simulink library "MBDS_Applications"  (R2018b)
settings: Solver=ode45  StartTime=0.0  StopTime=10.0  RelTol=1e-3
undefined symbols (not defined in the file or in its folder): Ts
libraries: KIBES_Signal x297, simulink x7
(part 4 of 6)

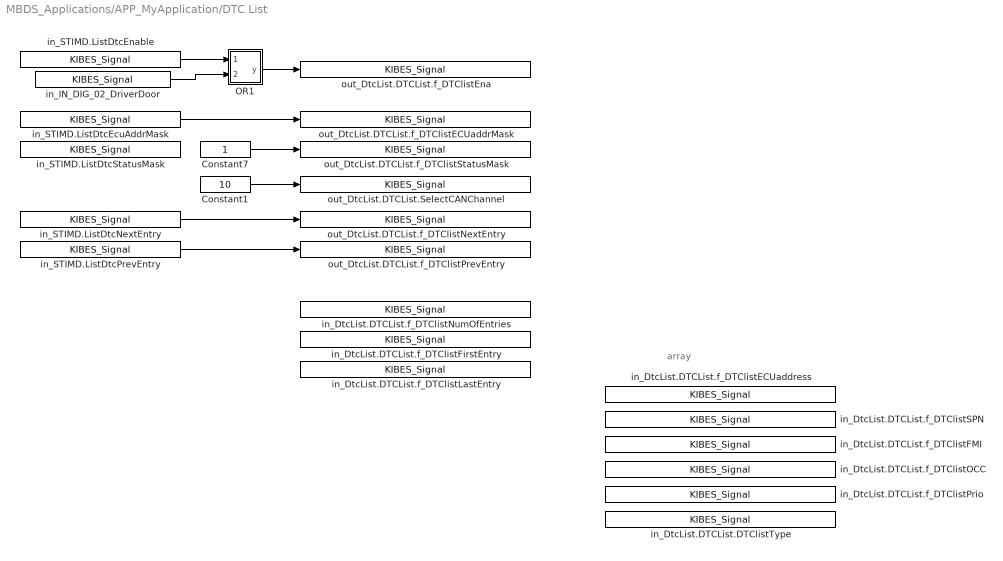
== system MBDS_Applications/APP_MyApplication/DTC List ==
  note: array
  Constant1 : Constant  InitFcn=|  Value=10  OutDataTypeStr=uint8
      | if(exist('MBDS_BlockCallback', 'file'))
      |    MBDS_BlockCallback('Update', gcb);  
      | end
  Constant7 : Constant  InitFcn=|  OutDataTypeStr=uint8
      | if(exist('MBDS_BlockCallback', 'file'))
      |    MBDS_BlockCallback('Update', gcb);  
      | end
  OR1 : Subsystem  InitFcn=|  mask(OR){MBDS_LibraryBlock=on, BitwiseMode=off, Inputs=2, UseBitMask=off, BitMask='A1', OutDataTypeStr=Inherit: Inherit via back propagation, MBDS_BlockVersion=07.21.05}
      | if(exist('MBDS_BlockCallback', 'file'))
      |    MBDS_BlockCallback('Update', gcb);
      | end
      mask prompts: MBDS_LibraryBlock "MBDS library block"; BitwiseMode "Use 'bitwise' mode"; Inputs "Number of input ports:"; UseBitMask "Use bit mask"; BitMask "Bit mask:"; OutDataTypeStr "Output data type:"; MBDS_BlockVersion "Version:"
      mask help: Logical or bitwise OR operator. For multiple inputs, operators are applied across the inputs. For a single input, operators are applied across the input vector. In bitwise mode a bit mask can be applied onto single input signals.
      mask init: same as MBDS_Applications/APP_MyApplication/NOT
      mask Help: eval(['open([workdir(''library_dir:''),''\Blockset\help\'',get_param(gcb,''MaskType''),''.html''])'])
      mask Callback BitwiseMode:
      | if(exist('MBDS_BlockCallback', 'file'))
      |    MBDS_BlockCallback('BitwiseMode', gcb);
      | end
      mask Callback Inputs:
      | if(exist('MBDS_BlockCallback', 'file'))
      |    MBDS_BlockCallback('Inputs', gcb);
      | end
      mask Callback UseBitMask:
      | if(exist('MBDS_BlockCallback', 'file'))
      |    MBDS_BlockCallback('UseBitMask', gcb);
      | end
      mask Callback BitMask:
      | if(exist('MBDS_BlockCallback', 'file'))
      |    MBDS_BlockCallback('BitMask', gcb);
      | end
      mask TypeOptions OutDataTypeStr: Inherit: Inherit via back propagation | int8 | uint8 | int16 | uint16 | int32 | uint32 | boolean
      mask Callback OutDataTypeStr:
      | % Adopt Value
      | if(exist('MBDS_BlockCallback', 'file'))
      |    MBDS_BlockCallback('OutDataTypeStr', gcb);
      | end
      mask DialogControl ParameterTabVar0 Prompt: Main
      mask DialogControl ParameterTabVar01 Prompt: Signal Attributes
      mask DialogControl ParameterTabVar012 Prompt: Version
      mask Display:
      | % Show icon or block text
      | if(UseBitMask)
      |    if(isnumeric(BitMask))
      |       BitMaskString = ['0x',dec2hex(floor(BitMask))];
      |    elseif(ischar(BitMask))
      |       BitMaskString = ['0x',upper(BitMask)];
      |    else
      |       BitMaskString = '???';
      |    end
      |    disp(sprintf(['OR\n', BitMaskString]))
      | else
      |    disp('OR')
      | end
  in_DtcList.DTCList.DTClistType : KIBES_Signal/KIBES_Signal  MBDS_LibraryBlock=on  DatabaseKey=268  SignalName=DtcList.DTCList.DTClistType  SymbolName=DtcList_DTCList_DTClistType_000268  DataType=uint8  Init=[0 0 0 0 0 0 0 0 0 0]  Slope=1  Bias=0  DataSize=10  fpDataType=uint8  BlockIOType=Inport  DeviceType=0
  in_DtcList.DTCList.f_DTClistECUaddress : KIBES_Signal/KIBES_Signal  MBDS_LibraryBlock=on  DatabaseKey=241  SignalName=DtcList.DTCList.f_DTClistECUaddress  SymbolName=DtcList_DTCList_f_DTClistECUaddress_000241  DataType=uint8  Init=[0 0 0 0 0 0 0 0 0 0]  Slope=1  Bias=0  DataSize=10  fpDataType=uint8  BlockIOType=Inport  DeviceType=0
  in_DtcList.DTCList.f_DTClistFMI : KIBES_Signal/KIBES_Signal  MBDS_LibraryBlock=on  DatabaseKey=245  SignalName=DtcList.DTCList.f_DTClistFMI  SymbolName=DtcList_DTCList_f_DTClistFMI_000245  DataType=uint8  Init=[0 0 0 0 0 0 0 0 0 0]  Slope=1  Bias=0  DataSize=10  fpDataType=uint8  BlockIOType=Inport  DeviceType=0
  in_DtcList.DTCList.f_DTClistFirstEntry : KIBES_Signal/KIBES_Signal  MBDS_LibraryBlock=on  DatabaseKey=244  SignalName=DtcList.DTCList.f_DTClistFirstEntry  SymbolName=DtcList_DTCList_f_DTClistFirstEntry_000244  DataType=boolean  Init=0  Slope=1  Bias=0  DataSize=1  fpDataType=boolean  BlockIOType=Inport  DeviceType=0
  in_DtcList.DTCList.f_DTClistLastEntry : KIBES_Signal/KIBES_Signal  MBDS_LibraryBlock=on  DatabaseKey=246  SignalName=DtcList.DTCList.f_DTClistLastEntry  SymbolName=DtcList_DTCList_f_DTClistLastEntry_000246  DataType=boolean  Init=0  Slope=1  Bias=0  DataSize=1  fpDataType=boolean  BlockIOType=Inport  DeviceType=0
  in_DtcList.DTCList.f_DTClistNumOfEntries : KIBES_Signal/KIBES_Signal  MBDS_LibraryBlock=on  DatabaseKey=248  SignalName=DtcList.DTCList.f_DTClistNumOfEntries  SymbolName=DtcList_DTCList_f_DTClistNumOfEntries_000248  DataType=uint16  Init=0  Slope=1  Bias=0  DataSize=1  fpDataType=uint16  BlockIOType=Inport  DeviceType=0
  in_DtcList.DTCList.f_DTClistOCC : KIBES_Signal/KIBES_Signal  MBDS_LibraryBlock=on  DatabaseKey=249  SignalName=DtcList.DTCList.f_DTClistOCC  SymbolName=DtcList_DTCList_f_DTClistOCC_000249  DataType=uint8  Init=[0 0 0 0 0 0 0 0 0 0]  Slope=1  Bias=0  DataSize=10  fpDataType=uint8  BlockIOType=Inport  DeviceType=0
  in_DtcList.DTCList.f_DTClistPrio : KIBES_Signal/KIBES_Signal  MBDS_LibraryBlock=on  DatabaseKey=251  SignalName=DtcList.DTCList.f_DTClistPrio  SymbolName=DtcList_DTCList_f_DTClistPrio_000251  DataType=uint8  Init=[0 0 0 0 0 0 0 0 0 0]  Slope=1  Bias=0  DataSize=10  fpDataType=uint8  BlockIOType=Inport  DeviceType=0
  in_DtcList.DTCList.f_DTClistSPN : KIBES_Signal/KIBES_Signal  MBDS_LibraryBlock=on  DatabaseKey=252  SignalName=DtcList.DTCList.f_DTClistSPN  SymbolName=DtcList_DTCList_f_DTClistSPN_000252  DataType=uint32  Init=[0 0 0 0 0 0 0 0 0 0]  Slope=1  Bias=0  DataSize=10  fpDataType=uint32  BlockIOType=Inport  DeviceType=0
  in_IN_DIG_02_DriverDoor : KIBES_Signal/KIBES_Signal  MBDS_LibraryBlock=on  DatabaseKey=215  SignalName=IN_DIG_02_DriverDoor  SymbolName=IN_DIG_02_DriverDoor_000215  DataType=boolean  Init=0  Slope=1  Bias=0  DataSize=1  fpDataType=boolean  BlockIOType=Inport  DeviceType=0
  in_STIMD.ListDtcEcuAddrMask : KIBES_Signal/KIBES_Signal  MBDS_LibraryBlock=on  DatabaseKey=254  SignalName=STIMD.ListDtcEcuAddrMask  SymbolName=STIMD_ListDtcEcuAddrMask_000254  DataType=uint8  Init=255  Slope=1  Bias=0  DataSize=1  fpDataType=uint8  BlockIOType=Inport  DeviceType=2
  in_STIMD.ListDtcEnable : KIBES_Signal/KIBES_Signal  MBDS_LibraryBlock=on  DatabaseKey=255  SignalName=STIMD.ListDtcEnable  SymbolName=STIMD_ListDtcEnable_000255  DataType=boolean  Init=0  Slope=1  Bias=0  DataSize=1  fpDataType=boolean  BlockIOType=Inport  DeviceType=2
  in_STIMD.ListDtcNextEntry : KIBES_Signal/KIBES_Signal  MBDS_LibraryBlock=on  DatabaseKey=256  SignalName=STIMD.ListDtcNextEntry  SymbolName=STIMD_ListDtcNextEntry_000256  DataType=boolean  Init=0  Slope=1  Bias=0  DataSize=1  fpDataType=boolean  BlockIOType=Inport  DeviceType=2
  in_STIMD.ListDtcPrevEntry : KIBES_Signal/KIBES_Signal  MBDS_LibraryBlock=on  DatabaseKey=257  SignalName=STIMD.ListDtcPrevEntry  SymbolName=STIMD_ListDtcPrevEntry_000257  DataType=boolean  Init=0  Slope=1  Bias=0  DataSize=1  fpDataType=boolean  BlockIOType=Inport  DeviceType=2
  in_STIMD.ListDtcStatusMask : KIBES_Signal/KIBES_Signal  MBDS_LibraryBlock=on  DatabaseKey=258  SignalName=STIMD.ListDtcStatusMask  SymbolName=STIMD_ListDtcStatusMask_000258  DataType=uint8  Init=255  Slope=1  Bias=0  DataSize=1  fpDataType=uint8  BlockIOType=Inport  DeviceType=2
  out_DtcList.DTCList.SelectCANChannel : KIBES_Signal/KIBES_Signal  MBDS_LibraryBlock=on  DatabaseKey=269  SignalName=DtcList.DTCList.SelectCANChannel  SymbolName=DtcList_DTCList_SelectCANChannel_000269  DataType=uint8  Init=0  Slope=1  Bias=0  DataSize=1  fpDataType=uint8  BlockIOType=Outport  DeviceType=0
  out_DtcList.DTCList.f_DTClistECUaddrMask : KIBES_Signal/KIBES_Signal  MBDS_LibraryBlock=on  DatabaseKey=242  SignalName=DtcList.DTCList.f_DTClistECUaddrMask  SymbolName=DtcList_DTCList_f_DTClistECUaddrMask_000242  DataType=uint8  Init=0  Slope=1  Bias=0  DataSize=1  fpDataType=uint8  BlockIOType=Outport  DeviceType=0
  out_DtcList.DTCList.f_DTClistEna : KIBES_Signal/KIBES_Signal  MBDS_LibraryBlock=on  DatabaseKey=243  SignalName=DtcList.DTCList.f_DTClistEna  SymbolName=DtcList_DTCList_f_DTClistEna_000243  DataType=boolean  Init=0  Slope=1  Bias=0  DataSize=1  fpDataType=boolean  BlockIOType=Outport  DeviceType=0
  out_DtcList.DTCList.f_DTClistNextEntry : KIBES_Signal/KIBES_Signal  MBDS_LibraryBlock=on  DatabaseKey=247  SignalName=DtcList.DTCList.f_DTClistNextEntry  SymbolName=DtcList_DTCList_f_DTClistNextEntry_000247  DataType=boolean  Init=0  Slope=1  Bias=0  DataSize=1  fpDataType=boolean  BlockIOType=Outport  DeviceType=0
  out_DtcList.DTCList.f_DTClistPrevEntry : KIBES_Signal/KIBES_Signal  MBDS_LibraryBlock=on  DatabaseKey=250  SignalName=DtcList.DTCList.f_DTClistPrevEntry  SymbolName=DtcList_DTCList_f_DTClistPrevEntry_000250  DataType=boolean  Init=0  Slope=1  Bias=0  DataSize=1  fpDataType=boolean  BlockIOType=Outport  DeviceType=0
  out_DtcList.DTCList.f_DTClistStatusMask : KIBES_Signal/KIBES_Signal  MBDS_LibraryBlock=on  DatabaseKey=253  SignalName=DtcList.DTCList.f_DTClistStatusMask  SymbolName=DtcList_DTCList_f_DTClistStatusMask_000253  DataType=uint8  Init=0  Slope=1  Bias=0  DataSize=1  fpDataType=uint8  BlockIOType=Outport  DeviceType=0
  wires:
  Constant1/1 -> out_DtcList.DTCList.SelectCANChannel/1
  Constant7/1 -> out_DtcList.DTCList.f_DTClistStatusMask/1
  in_IN_DIG_02_DriverDoor/1 -> OR1/2(u2)
  in_STIMD.ListDtcEnable/1 -> OR1/1(u1)
  OR1/1(y) -> out_DtcList.DTCList.f_DTClistEna/1
  in_STIMD.ListDtcPrevEntry/1 -> out_DtcList.DTCList.f_DTClistPrevEntry/1
  in_STIMD.ListDtcNextEntry/1 -> out_DtcList.DTCList.f_DTClistNextEntry/1
  in_STIMD.ListDtcEcuAddrMask/1 -> out_DtcList.DTCList.f_DTClistECUaddrMask/1

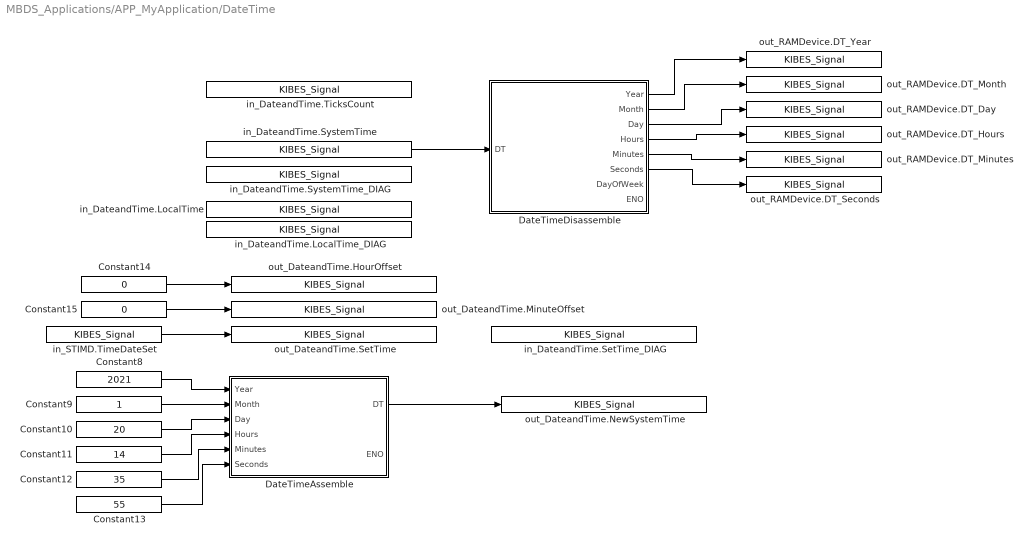
== system MBDS_Applications/APP_MyApplication/DateTime ==
  Constant10 : Constant  InitFcn=|  Value=20  OutDataTypeStr=uint8
      | if(exist('MBDS_BlockCallback', 'file'))
      |    MBDS_BlockCallback('Update', gcb);  
      | end
  Constant11 : Constant  InitFcn=|  Value=14  OutDataTypeStr=uint8
      | if(exist('MBDS_BlockCallback', 'file'))
      |    MBDS_BlockCallback('Update', gcb);  
      | end
  Constant12 : Constant  InitFcn=|  Value=35  OutDataTypeStr=uint8
      | if(exist('MBDS_BlockCallback', 'file'))
      |    MBDS_BlockCallback('Update', gcb);  
      | end
  Constant13 : Constant  InitFcn=|  Value=55  OutDataTypeStr=uint8
      | if(exist('MBDS_BlockCallback', 'file'))
      |    MBDS_BlockCallback('Update', gcb);  
      | end
  Constant14 : Constant  InitFcn=|  Value=0  OutDataTypeStr=int8
      | if(exist('MBDS_BlockCallback', 'file'))
      |    MBDS_BlockCallback('Update', gcb);  
      | end
  Constant15 : Constant  InitFcn=|  Value=0  OutDataTypeStr=int8
      | if(exist('MBDS_BlockCallback', 'file'))
      |    MBDS_BlockCallback('Update', gcb);  
      | end
  Constant8 : Constant  InitFcn=|  Value=2021  OutDataTypeStr=uint16
      | if(exist('MBDS_BlockCallback', 'file'))
      |    MBDS_BlockCallback('Update', gcb);  
      | end
  Constant9 : Constant  InitFcn=|  OutDataTypeStr=uint8
      | if(exist('MBDS_BlockCallback', 'file'))
      |    MBDS_BlockCallback('Update', gcb);  
      | end
  DateTimeAssemble : Subsystem  mask(DateTimeAssemble){MBDS_LibraryBlock=on, ENO_Enabled=on, MBDS_BlockVersion=07.21.06}
      mask prompts: MBDS_LibraryBlock "MBDS library block"; ENO_Enabled "Show ENO port"; MBDS_BlockVersion "Block version:"
      mask help: Assembles a date_time signal from individual date and time components. The input values are restricted to their ranges (refer to the block help). If an input is out of range the ENO output is set to false.
      mask init: same as MBDS_Applications/APP_MyApplication/NOT
      mask Help: eval(['open([workdir(''Library_Dir:''),''\Blockset\Help\'',get_param(gcb,''MaskType''),''.html''])']);
      mask DialogControl Container4 Prompt: Main
      mask DialogControl Container5 Prompt: Version
      mask Display:
      | % Show block text
      | disp(sprintf('DateTime\nAssemble'));
      | 
      | % Display port labels
      | port_label('input', 1, 'Year');
      | port_label('input', 2, 'Month');
      | port_label('input', 3, 'Day');
      | port_label('input', 4, 'Hours');
      | port_label('input', 5, 'Minutes');
      | port_label('input', 6, 'Seconds');
      | port_label('output', 1, 'DT');
      | port_label('output', 2, 'ENO');
  DateTimeDisassemble : Subsystem  mask(DateTimeDisassemble){MBDS_LibraryBlock=on, ENO_Enabled=on, MBDS_BlockVersion=07.21.06}
      mask prompts: MBDS_LibraryBlock "MBDS library block"; ENO_Enabled "Show ENO port"; MBDS_BlockVersion "Block version:"
      mask help: Disassembles a date_time signal into its date time components, i.e. year, month, day, hour, minute, second. Additionally the day of week number is output. If the input signal is invalid the ENO output is false.
      mask init: same as MBDS_Applications/APP_MyApplication/NOT
      mask Help: eval(['open([workdir(''Library_Dir:''),''\Blockset\Help\'',get_param(gcb,''MaskType''),''.html''])']);
      mask DialogControl Container8 Prompt: Main
      mask DialogControl Container11 Prompt: Version
      mask Display:
      | % Show block text
      | disp(sprintf('DateTime\nDisassemble'));
      | 
      | % Display port labels
      | port_label('input', 1, 'DT');
      | port_label('output', 1, 'Year');
      | port_label('output', 2, 'Month');
      | port_label('output', 3, 'Day');
      | port_label('output', 4, 'Hours');
      | port_label('output', 5, 'Minutes');
      | port_label('output', 6, 'Seconds');
      | port_label('output', 7, 'DayOfWeek');
      | port_label('output', 8, 'ENO');
  in_DateandTime.LocalTime : KIBES_Signal/KIBES_Signal  MBDS_LibraryBlock=on  DatabaseKey=415  SignalName=DateandTime.LocalTime  SymbolName=DateandTime_LocalTime_000415  DataType=uint32  Init=0  Slope=1  Bias=0  DataSize=1  fpDataType=uint32  BlockIOType=Inport  DeviceType=0
  in_DateandTime.LocalTime_DIAG : KIBES_Signal/KIBES_Signal  MBDS_LibraryBlock=on  DatabaseKey=418  SignalName=DateandTime.LocalTime_DIAG  SymbolName=DateandTime_LocalTime_DIAG_000418  DataType=uint16  Init=1  Slope=1  Bias=0  DataSize=1  fpDataType=uint16  BlockIOType=Inport  DeviceType=0
  in_DateandTime.SetTime_DIAG : KIBES_Signal/KIBES_Signal  MBDS_LibraryBlock=on  DatabaseKey=410  SignalName=DateandTime.SetTime_DIAG  SymbolName=DateandTime_SetTime_DIAG_000410  DataType=uint16  Init=1  Slope=1  Bias=0  DataSize=1  fpDataType=uint16  BlockIOType=Inport  DeviceType=0
  in_DateandTime.SystemTime : KIBES_Signal/KIBES_Signal  MBDS_LibraryBlock=on  DatabaseKey=412  SignalName=DateandTime.SystemTime  SymbolName=DateandTime_SystemTime_000412  DataType=uint32  Init=0  Slope=1  Bias=0  DataSize=1  fpDataType=uint32  BlockIOType=Inport  DeviceType=0
  in_DateandTime.SystemTime_DIAG : KIBES_Signal/KIBES_Signal  MBDS_LibraryBlock=on  DatabaseKey=413  SignalName=DateandTime.SystemTime_DIAG  SymbolName=DateandTime_SystemTime_DIAG_000413  DataType=uint16  Init=1  Slope=1  Bias=0  DataSize=1  fpDataType=uint16  BlockIOType=Inport  DeviceType=0
  in_DateandTime.TicksCount : KIBES_Signal/KIBES_Signal  MBDS_LibraryBlock=on  DatabaseKey=414  SignalName=DateandTime.TicksCount  SymbolName=DateandTime_TicksCount_000414  DataType=uint32  Init=0  Slope=1  Bias=0  DataSize=1  fpDataType=uint32  BlockIOType=Inport  DeviceType=0
  in_STIMD.TimeDateSet : KIBES_Signal/KIBES_Signal  MBDS_LibraryBlock=on  DatabaseKey=420  SignalName=STIMD.TimeDateSet  SymbolName=STIMD_TimeDateSet_000420  DataType=boolean  Init=0  Slope=1  Bias=0  DataSize=1  fpDataType=boolean  BlockIOType=Inport  DeviceType=2
  out_DateandTime.HourOffset : KIBES_Signal/KIBES_Signal  MBDS_LibraryBlock=on  DatabaseKey=416  SignalName=DateandTime.HourOffset  SymbolName=DateandTime_HourOffset_000416  DataType=int8  Init=0  Slope=1  Bias=0  DataSize=1  fpDataType=int8  BlockIOType=Outport  DeviceType=0
  out_DateandTime.MinuteOffset : KIBES_Signal/KIBES_Signal  MBDS_LibraryBlock=on  DatabaseKey=419  SignalName=DateandTime.MinuteOffset  SymbolName=DateandTime_MinuteOffset_000419  DataType=int8  Init=0  Slope=1  Bias=0  DataSize=1  fpDataType=int8  BlockIOType=Outport  DeviceType=0
  out_DateandTime.NewSystemTime : KIBES_Signal/KIBES_Signal  MBDS_LibraryBlock=on  DatabaseKey=417  SignalName=DateandTime.NewSystemTime  SymbolName=DateandTime_NewSystemTime_000417  DataType=uint32  Init=0  Slope=1  Bias=0  DataSize=1  fpDataType=uint32  BlockIOType=Outport  DeviceType=0
  out_DateandTime.SetTime : KIBES_Signal/KIBES_Signal  MBDS_LibraryBlock=on  DatabaseKey=411  SignalName=DateandTime.SetTime  SymbolName=DateandTime_SetTime_000411  DataType=boolean  Init=0  Slope=1  Bias=0  DataSize=1  fpDataType=boolean  BlockIOType=Outport  DeviceType=0
  out_RAMDevice.DT_Day : KIBES_Signal/KIBES_Signal  MBDS_LibraryBlock=on  DatabaseKey=424  SignalName=RAMDevice.DT_Day  SymbolName=RAMDevice_DT_Day_000424  DataType=uint8  Init=0  Slope=1  Bias=0  DataSize=1  fpDataType=uint8  BlockIOType=Outport  DeviceType=0
  out_RAMDevice.DT_Hours : KIBES_Signal/KIBES_Signal  MBDS_LibraryBlock=on  DatabaseKey=423  SignalName=RAMDevice.DT_Hours  SymbolName=RAMDevice_DT_Hours_000423  DataType=uint8  Init=0  Slope=1  Bias=0  DataSize=1  fpDataType=uint8  BlockIOType=Outport  DeviceType=0
  out_RAMDevice.DT_Minutes : KIBES_Signal/KIBES_Signal  MBDS_LibraryBlock=on  DatabaseKey=425  SignalName=RAMDevice.DT_Minutes  SymbolName=RAMDevice_DT_Minutes_000425  DataType=uint8  Init=0  Slope=1  Bias=0  DataSize=1  fpDataType=uint8  BlockIOType=Outport  DeviceType=0
  out_RAMDevice.DT_Month : KIBES_Signal/KIBES_Signal  MBDS_LibraryBlock=on  DatabaseKey=422  SignalName=RAMDevice.DT_Month  SymbolName=RAMDevice_DT_Month_000422  DataType=uint8  Init=0  Slope=1  Bias=0  DataSize=1  fpDataType=uint8  BlockIOType=Outport  DeviceType=0
  out_RAMDevice.DT_Seconds : KIBES_Signal/KIBES_Signal  MBDS_LibraryBlock=on  DatabaseKey=426  SignalName=RAMDevice.DT_Seconds  SymbolName=RAMDevice_DT_Seconds_000426  DataType=uint8  Init=0  Slope=1  Bias=0  DataSize=1  fpDataType=uint8  BlockIOType=Outport  DeviceType=0
  out_RAMDevice.DT_Year : KIBES_Signal/KIBES_Signal  MBDS_LibraryBlock=on  DatabaseKey=421  SignalName=RAMDevice.DT_Year  SymbolName=RAMDevice_DT_Year_000421  DataType=uint16  Init=0  Slope=1  Bias=0  DataSize=1  fpDataType=uint16  BlockIOType=Outport  DeviceType=0
  wires:
  DateTimeDisassemble/6(Seconds) -> out_RAMDevice.DT_Seconds/1
  DateTimeDisassemble/3(Day) -> out_RAMDevice.DT_Day/1
  DateTimeDisassemble/4(Hours) -> out_RAMDevice.DT_Hours/1
  DateTimeDisassemble/5(Minutes) -> out_RAMDevice.DT_Minutes/1
  DateTimeDisassemble/1(Year) -> out_RAMDevice.DT_Year/1
  DateTimeDisassemble/2(Month) -> out_RAMDevice.DT_Month/1
  in_DateandTime.SystemTime/1 -> DateTimeDisassemble/1(DT)
  in_STIMD.TimeDateSet/1 -> out_DateandTime.SetTime/1
  Constant15/1 -> out_DateandTime.MinuteOffset/1
  Constant14/1 -> out_DateandTime.HourOffset/1
  Constant13/1 -> DateTimeAssemble/6(Seconds)
  Constant12/1 -> DateTimeAssemble/5(Minutes)
  Constant11/1 -> DateTimeAssemble/4(Hours)
  Constant10/1 -> DateTimeAssemble/3(Day)
  Constant9/1 -> DateTimeAssemble/2(Month)
  Constant8/1 -> DateTimeAssemble/1(Year)
  DateTimeAssemble/1(DT) -> out_DateandTime.NewSystemTime/1

== system MBDS_Applications/APP_MyApplication/EEProm ==
  note: Variable DID 0x125 and size 4 byte / access in extended session 03 and level 3
      | EEProm layout 4Bytes: VarB0, VarU16
      | Default value: True 1234=0x04D2
      | UDS command Read 22 01 25
      | UDS command Write 2E 01 25 01 00 22 33
  note: Parameter DID 0x123 and size 5 byte / access in extended session 03 and level 3
      | EEProm layout Bytes: byte, u16, u16 (complete structure does use 6 bytes)
      | Default value: 1 2 3
      | UDS command Write 2E 01 23 01 02 03 04 05 06
      | Displayed in CAN message 0x18030121 00 00 01 00 04 03 06 05
      | Device state 08 01 if EEPROM does use default values, all CAN values are u16
  Constant8 : Constant  InitFcn=|  Value=0  OutDataTypeStr=boolean
      | if(exist('MBDS_BlockCallback', 'file'))
      |    MBDS_BlockCallback('Update', gcb);  
      | end
  Constant9 : Constant  InitFcn=|  Value=0  OutDataTypeStr=boolean
      | if(exist('MBDS_BlockCallback', 'file'))
      |    MBDS_BlockCallback('Update', gcb);  
      | end
  Data Type Conversion : DataTypeConversion  InitFcn=|  SaturateOnIntegerOverflow=on
      | try
      |    MBDS_BlockCallback('Update', gcb);
      | end
      settings: AttributesFormatString=Saturate: %<SaturateOnIntegerOverflow>
  Data Type Conversion1 : DataTypeConversion  InitFcn=|  SaturateOnIntegerOverflow=on
      | try
      |    MBDS_BlockCallback('Update', gcb);
      | end
      settings: AttributesFormatString=Saturate: %<SaturateOnIntegerOverflow>
  in_NVMModelRelatedData.NVMParameter.DeviceState : KIBES_Signal/KIBES_Signal  MBDS_LibraryBlock=on  DatabaseKey=167  SignalName=NVMModelRelatedData.NVMParameter.DeviceState  SymbolName=NVMModelRelatedData_NVMParameter_DeviceState_000167  DataType=uint16  Init=0  Slope=1  Bias=0  DataSize=1  fpDataType=uint16  BlockIOType=Inport  DeviceType=0
  in_NVMModelRelatedData.NVMParameter.Variable_00 : KIBES_Signal/KIBES_Signal  MBDS_LibraryBlock=on  DatabaseKey=168  SignalName=NVMModelRelatedData.NVMParameter.Variable_00  SymbolName=NVMModelRelatedData_NVMParameter_Variable_00_000168  DataType=uint8  Init=1  Slope=1  Bias=0  DataSize=1  fpDataType=uint8  BlockIOType=Inport  DeviceType=0
  in_NVMModelRelatedData.NVMParameter.Variable_01 : KIBES_Signal/KIBES_Signal  MBDS_LibraryBlock=on  DatabaseKey=169  SignalName=NVMModelRelatedData.NVMParameter.Variable_01  SymbolName=NVMModelRelatedData_NVMParameter_Variable_01_000169  DataType=uint16  Init=2  Slope=1  Bias=0  DataSize=1  fpDataType=uint16  BlockIOType=Inport  DeviceType=0
  in_NVMModelRelatedData.NVMParameter.Variable_02 : KIBES_Signal/KIBES_Signal  MBDS_LibraryBlock=on  DatabaseKey=170  SignalName=NVMModelRelatedData.NVMParameter.Variable_02  SymbolName=NVMModelRelatedData_NVMParameter_Variable_02_000170  DataType=uint16  Init=3  Slope=1  Bias=0  DataSize=1  fpDataType=uint16  BlockIOType=Inport  DeviceType=0
  in_NVMModelRelatedData.NVMVariables.DeviceState : KIBES_Signal/KIBES_Signal  MBDS_LibraryBlock=on  DatabaseKey=160  SignalName=NVMModelRelatedData.NVMVariables.DeviceState  SymbolName=NVMModelRelatedData_NVMVariables_DeviceState_000160  DataType=uint16  Init=0  Slope=1  Bias=0  DataSize=1  fpDataType=uint16  BlockIOType=Inport  DeviceType=0
  in_NVMModelRelatedData.NVMVariables.Variable_bo : KIBES_Signal/KIBES_Signal  MBDS_LibraryBlock=on  DatabaseKey=161  SignalName=NVMModelRelatedData.NVMVariables.Variable_bo  SymbolName=NVMModelRelatedData_NVMVariables_Variable_bo_000161  DataType=boolean  Init=1  Slope=1  Bias=0  DataSize=1  fpDataType=boolean  BlockIOType=Inport  DeviceType=0
  in_NVMModelRelatedData.NVMVariables.Variable_u16 : KIBES_Signal/KIBES_Signal  MBDS_LibraryBlock=on  DatabaseKey=162  SignalName=NVMModelRelatedData.NVMVariables.Variable_u16  SymbolName=NVMModelRelatedData_NVMVariables_Variable_u16_000162  DataType=uint16  Init=1234  Slope=1  Bias=0  DataSize=1  fpDataType=uint16  BlockIOType=Inport  DeviceType=0
  out_DCAN.TX_Gen.DGenTX_2.MessageEnable : KIBES_Signal/KIBES_Signal  MBDS_LibraryBlock=on  DatabaseKey=163  SignalName=DCAN.TX_Gen.DGenTX_2.MessageEnable  SymbolName=DCAN_TX_Gen_DGenTX_2_MessageEnable_000163  DataType=boolean  Init=0  Slope=1  Bias=0  DataSize=1  fpDataType=boolean  BlockIOType=Outport  DeviceType=0
  out_DCAN.TX_Gen.DGenTX_2.Val1 : KIBES_Signal/KIBES_Signal  MBDS_LibraryBlock=on  DatabaseKey=164  SignalName=DCAN.TX_Gen.DGenTX_2.Val1  SymbolName=DCAN_TX_Gen_DGenTX_2_Val1_000164  DataType=uint16  Init=0  Slope=1  Bias=0  DataSize=1  fpDataType=uint16  BlockIOType=Outport  DeviceType=0
  out_DCAN.TX_Gen.DGenTX_2.Val2 : KIBES_Signal/KIBES_Signal  MBDS_LibraryBlock=on  DatabaseKey=165  SignalName=DCAN.TX_Gen.DGenTX_2.Val2  SymbolName=DCAN_TX_Gen_DGenTX_2_Val2_000165  DataType=uint16  Init=0  Slope=1  Bias=0  DataSize=1  fpDataType=uint16  BlockIOType=Outport  DeviceType=0
  out_DCAN.TX_Gen.DGenTX_2.Val3 : KIBES_Signal/KIBES_Signal  MBDS_LibraryBlock=on  DatabaseKey=166  SignalName=DCAN.TX_Gen.DGenTX_2.Val3  SymbolName=DCAN_TX_Gen_DGenTX_2_Val3_000166  DataType=uint16  Init=0  Slope=1  Bias=0  DataSize=1  fpDataType=uint16  BlockIOType=Outport  DeviceType=0
  out_DCAN.TX_Gen.DGenTX_3.MessageEnable : KIBES_Signal/KIBES_Signal  MBDS_LibraryBlock=on  DatabaseKey=171  SignalName=DCAN.TX_Gen.DGenTX_3.MessageEnable  SymbolName=DCAN_TX_Gen_DGenTX_3_MessageEnable_000171  DataType=boolean  Init=0  Slope=1  Bias=0  DataSize=1  fpDataType=boolean  BlockIOType=Outport  DeviceType=0
  out_DCAN.TX_Gen.DGenTX_3.Val1 : KIBES_Signal/KIBES_Signal  MBDS_LibraryBlock=on  DatabaseKey=172  SignalName=DCAN.TX_Gen.DGenTX_3.Val1  SymbolName=DCAN_TX_Gen_DGenTX_3_Val1_000172  DataType=uint16  Init=0  Slope=1  Bias=0  DataSize=1  fpDataType=uint16  BlockIOType=Outport  DeviceType=0
  out_DCAN.TX_Gen.DGenTX_3.Val2 : KIBES_Signal/KIBES_Signal  MBDS_LibraryBlock=on  DatabaseKey=173  SignalName=DCAN.TX_Gen.DGenTX_3.Val2  SymbolName=DCAN_TX_Gen_DGenTX_3_Val2_000173  DataType=uint16  Init=0  Slope=1  Bias=0  DataSize=1  fpDataType=uint16  BlockIOType=Outport  DeviceType=0
  out_DCAN.TX_Gen.DGenTX_3.Val3 : KIBES_Signal/KIBES_Signal  MBDS_LibraryBlock=on  DatabaseKey=174  SignalName=DCAN.TX_Gen.DGenTX_3.Val3  SymbolName=DCAN_TX_Gen_DGenTX_3_Val3_000174  DataType=uint16  Init=0  Slope=1  Bias=0  DataSize=1  fpDataType=uint16  BlockIOType=Outport  DeviceType=0
  out_DCAN.TX_Gen.DGenTX_3.Val4 : KIBES_Signal/KIBES_Signal  MBDS_LibraryBlock=on  DatabaseKey=175  SignalName=DCAN.TX_Gen.DGenTX_3.Val4  SymbolName=DCAN_TX_Gen_DGenTX_3_Val4_000175  DataType=uint16  Init=0  Slope=1  Bias=0  DataSize=1  fpDataType=uint16  BlockIOType=Outport  DeviceType=0
  wires:
  Constant9/1 -> out_DCAN.TX_Gen.DGenTX_3.MessageEnable/1
  Constant8/1 -> out_DCAN.TX_Gen.DGenTX_2.MessageEnable/1
  in_NVMModelRelatedData.NVMVariables.DeviceState/1 -> out_DCAN.TX_Gen.DGenTX_2.Val1/1
  in_NVMModelRelatedData.NVMParameter.Variable_00/1 -> Data Type Conversion1/1
  Data Type Conversion/1 -> out_DCAN.TX_Gen.DGenTX_2.Val2/1
  in_NVMModelRelatedData.NVMParameter.DeviceState/1 -> out_DCAN.TX_Gen.DGenTX_3.Val1/1
  in_NVMModelRelatedData.NVMVariables.Variable_bo/1 -> Data Type Conversion/1
  Data Type Conversion1/1 -> out_DCAN.TX_Gen.DGenTX_3.Val2/1
  in_NVMModelRelatedData.NVMParameter.Variable_02/1 -> out_DCAN.TX_Gen.DGenTX_3.Val4/1
  in_NVMModelRelatedData.NVMParameter.Variable_01/1 -> out_DCAN.TX_Gen.DGenTX_3.Val3/1
  in_NVMModelRelatedData.NVMVariables.Variable_u16/1 -> out_DCAN.TX_Gen.DGenTX_2.Val3/1

== system MBDS_Applications/APP_MyApplication/FMS-CAN ==
  note: 18010521
  Constant1 : Constant  InitFcn=|  Value=55  OutDataTypeStr=uint8
      | if(exist('MBDS_BlockCallback', 'file'))
      |    MBDS_BlockCallback('Update', gcb);  
      | end
  Constant3 : Constant  InitFcn=|  OutDataTypeStr=boolean
      | if(exist('MBDS_BlockCallback', 'file'))
      |    MBDS_BlockCallback('Update', gcb);  
      | end
  in_FMSCAN.TX_GEN.FMSGenTX_1.MessageState : KIBES_Signal/KIBES_Signal  MBDS_LibraryBlock=on  DatabaseKey=298  SignalName=FMSCAN.TX_GEN.FMSGenTX_1.MessageState  SymbolName=FMSCAN_TX_GEN_FMSGenTX_1_MessageState_000298  DataType=uint16  Init=0  Slope=1  Bias=0  DataSize=1  fpDataType=uint16  BlockIOType=Inport  DeviceType=0
  out_FMSCAN.TX_GEN.FMSGenTX_1.MessageEnable : KIBES_Signal/KIBES_Signal  MBDS_LibraryBlock=on  DatabaseKey=297  SignalName=FMSCAN.TX_GEN.FMSGenTX_1.MessageEnable  SymbolName=FMSCAN_TX_GEN_FMSGenTX_1_MessageEnable_000297  DataType=boolean  Init=0  Slope=1  Bias=0  DataSize=1  fpDataType=boolean  BlockIOType=Outport  DeviceType=0
  out_FMSCAN.TX_GEN.FMSGenTX_1.Val_1 : KIBES_Signal/KIBES_Signal  MBDS_LibraryBlock=on  DatabaseKey=299  SignalName=FMSCAN.TX_GEN.FMSGenTX_1.Val_1  SymbolName=FMSCAN_TX_GEN_FMSGenTX_1_Val_1_000299  DataType=uint8  Init=0  Slope=1  Bias=0  DataSize=1  fpDataType=uint8  BlockIOType=Outport  DeviceType=0
  wires:
  Constant1/1 -> out_FMSCAN.TX_GEN.FMSGenTX_1.Val_1/1
  Constant3/1 -> out_FMSCAN.TX_GEN.FMSGenTX_1.MessageEnable/1

== system MBDS_Applications/APP_MyApplication/H-CAN 500kBaud ==
  Constant1 : Constant  InitFcn=|  OutDataTypeStr=uint8
      | if(exist('MBDS_BlockCallback', 'file'))
      |    MBDS_BlockCallback('Update', gcb);  
      | end
  Constant2 : Constant  InitFcn=|  Value=2  OutDataTypeStr=uint8
      | if(exist('MBDS_BlockCallback', 'file'))
      |    MBDS_BlockCallback('Update', gcb);  
      | end
  Constant7 : Constant  InitFcn=|  OutDataTypeStr=boolean
      | if(exist('MBDS_BlockCallback', 'file'))
      |    MBDS_BlockCallback('Update', gcb);  
      | end
  in_HCAN.TX_GEN.HGenTX_1.MessageState : KIBES_Signal/KIBES_Signal  MBDS_LibraryBlock=on  DatabaseKey=265  SignalName=HCAN.TX_GEN.HGenTX_1.MessageState  SymbolName=HCAN_TX_GEN_HGenTX_1_MessageState_000265  DataType=uint16  Init=0  Slope=1  Bias=0  DataSize=1  fpDataType=uint16  BlockIOType=Inport  DeviceType=0
  out_HCAN.TX_GEN.HGenTX_1.MessageEnable : KIBES_Signal/KIBES_Signal  MBDS_LibraryBlock=on  DatabaseKey=264  SignalName=HCAN.TX_GEN.HGenTX_1.MessageEnable  SymbolName=HCAN_TX_GEN_HGenTX_1_MessageEnable_000264  DataType=boolean  Init=0  Slope=1  Bias=0  DataSize=1  fpDataType=boolean  BlockIOType=Outport  DeviceType=0
  out_HCAN.TX_GEN.HGenTX_1.Val_1 : KIBES_Signal/KIBES_Signal  MBDS_LibraryBlock=on  DatabaseKey=266  SignalName=HCAN.TX_GEN.HGenTX_1.Val_1  SymbolName=HCAN_TX_GEN_HGenTX_1_Val_1_000266  DataType=uint8  Init=0  Slope=1  Bias=0  DataSize=1  fpDataType=uint8  BlockIOType=Outport  DeviceType=0
  out_HCAN.TX_GEN.HGenTX_1.Val_2 : KIBES_Signal/KIBES_Signal  MBDS_LibraryBlock=on  DatabaseKey=267  SignalName=HCAN.TX_GEN.HGenTX_1.Val_2  SymbolName=HCAN_TX_GEN_HGenTX_1_Val_2_000267  DataType=uint8  Init=0  Slope=1  Bias=0  DataSize=1  fpDataType=uint8  BlockIOType=Outport  DeviceType=0
  wires:
  Constant2/1 -> out_HCAN.TX_GEN.HGenTX_1.Val_2/1
  Constant1/1 -> out_HCAN.TX_GEN.HGenTX_1.Val_1/1
  Constant7/1 -> out_HCAN.TX_GEN.HGenTX_1.MessageEnable/1

== system MBDS_Applications/APP_MyApplication/NOT ==
  note: NOT
  u1 : Inport  OutDataTypeStr=boolean
  DataType : DataTypeConversion  OutDataTypeStr=boolean
  Operator : Logic  Operator=NOT  Inputs=1  AllPortsSameDT=off  OutDataTypeStr=boolean
  y : Outport
  wires:
  DataType/1 -> y/1
  u1/1 -> Operator/1
  Operator/1 -> DataType/1

== system MBDS_Applications/APP_MyApplication/OR ==
  note: OR
  u1 : Inport  OutDataTypeStr=boolean
  u2 : Inport  Port=2  OutDataTypeStr=boolean
  u3 : Inport  Port=3  OutDataTypeStr=boolean
  u4 : Inport  Port=4  OutDataTypeStr=boolean
  DataType : DataTypeConversion  OutDataTypeStr=boolean
  Operator : Logic  Operator=OR  Inputs=4  AllPortsSameDT=off  OutDataTypeStr=boolean
  y : Outport
  wires:
  u4/1 -> Operator/4
  u3/1 -> Operator/3
  DataType/1 -> y/1
  u2/1 -> Operator/2
  u1/1 -> Operator/1
  Operator/1 -> DataType/1

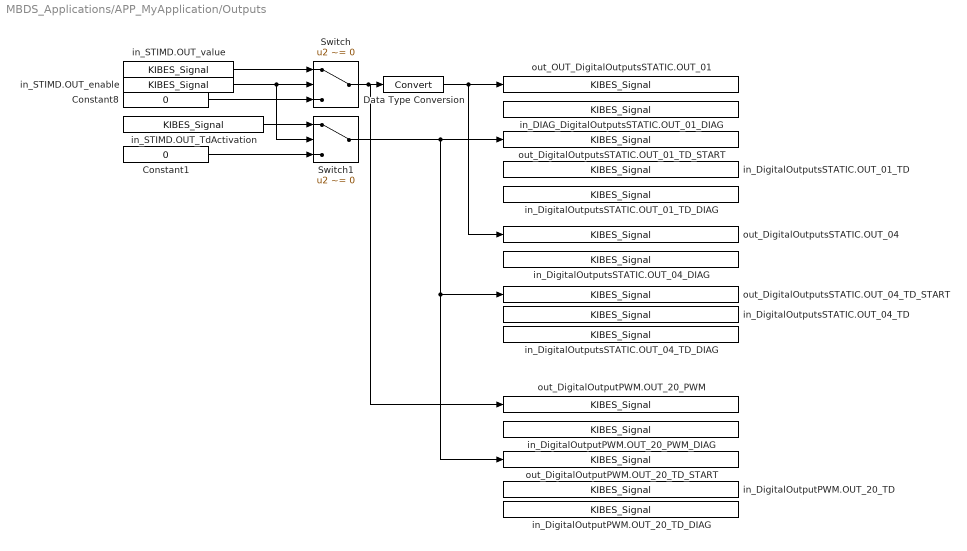
== system MBDS_Applications/APP_MyApplication/Outputs ==
  Constant1 : Constant  InitFcn=|  Value=0  OutDataTypeStr=uint8
      | if(exist('MBDS_BlockCallback', 'file'))
      |    MBDS_BlockCallback('Update', gcb);  
      | end
  Constant8 : Constant  InitFcn=|  Value=0  OutDataTypeStr=uint8
      | if(exist('MBDS_BlockCallback', 'file'))
      |    MBDS_BlockCallback('Update', gcb);  
      | end
  Data Type Conversion : DataTypeConversion  InitFcn=|  SaturateOnIntegerOverflow=on
      | try
      |    MBDS_BlockCallback('Update', gcb);
      | end
      settings: AttributesFormatString=Saturate: %<SaturateOnIntegerOverflow>
  Switch : Switch  InitFcn=|  Criteria=u2 ~= 0  OutDataTypeStr=Inherit: Inherit via back propagation  mask(Switch){MBDS_LibraryBlock=on, OutDataTypeStr_=Inherit: Inherit via back propagation, SaturateOnIntegerOverflow_=off, InputSameDT_=off, MBDS_BlockVersion=07.21.05}
      | if(exist('MBDS_BlockCallback', 'file'))
      |    MBDS_BlockCallback('Update', gcb);  
      | end
      mask prompts: MBDS_LibraryBlock "MBDS library block"; OutDataTypeStr_ "Output data type:"; SaturateOnIntegerOverflow_ "Saturate on integer overflow"; InputSameDT_ "Require all inputs to have the same data type"; MBDS_BlockVersion "Block version:"
      mask help: Pass through input 1 when input 2 is not equal to zero; otherwise pass through input 3. The inputs are numbered top to bottom (or left to right). The first and third input ports are data ports, and the second input port is the control port.
      mask init: same as MBDS_Applications/APP_MyApplication/NOT
      mask Help: eval(['open([workdir(''library_dir:''),''\Blockset\help\'',get_param(gcb,''MaskType''),''.html''])'])
      mask TypeOptions OutDataTypeStr_: Inherit: Inherit via back propagation | single | int8 | uint8 | int16 | uint16 | int32 | uint32
      mask DialogControl ParameterTabVar0 Prompt: Signal Attributes
      mask DialogControl ParameterTabVar01 Prompt: Version
  Switch1 : Switch  InitFcn=|  Criteria=u2 ~= 0  OutDataTypeStr=Inherit: Inherit via back propagation  mask(Switch){MBDS_LibraryBlock=on, OutDataTypeStr_=Inherit: Inherit via back propagation, SaturateOnIntegerOverflow_=off, InputSameDT_=off, MBDS_BlockVersion=07.21.05}
      | if(exist('MBDS_BlockCallback', 'file'))
      |    MBDS_BlockCallback('Update', gcb);  
      | end
      mask prompts: MBDS_LibraryBlock "MBDS library block"; OutDataTypeStr_ "Output data type:"; SaturateOnIntegerOverflow_ "Saturate on integer overflow"; InputSameDT_ "Require all inputs to have the same data type"; MBDS_BlockVersion "Block version:"
      mask help: Pass through input 1 when input 2 is not equal to zero; otherwise pass through input 3. The inputs are numbered top to bottom (or left to right). The first and third input ports are data ports, and the second input port is the control port.
      mask init: same as MBDS_Applications/APP_MyApplication/NOT
      mask Help: eval(['open([workdir(''library_dir:''),''\Blockset\help\'',get_param(gcb,''MaskType''),''.html''])'])
      mask TypeOptions OutDataTypeStr_: Inherit: Inherit via back propagation | single | int8 | uint8 | int16 | uint16 | int32 | uint32
      mask DialogControl ParameterTabVar0 Prompt: Signal Attributes
      mask DialogControl ParameterTabVar01 Prompt: Version
  in_DIAG_DigitalOutputsSTATIC.OUT_01_DIAG : KIBES_Signal/KIBES_Signal  MBDS_LibraryBlock=on  DatabaseKey=82  SignalName=DIAG_DigitalOutputsSTATIC.OUT_01_DIAG  SymbolName=DIAG_DigitalOutputsSTATIC_OUT_01_DIAG_000082  DataType=uint16  Init=1  Slope=1  Bias=0  DataSize=1  fpDataType=uint16  BlockIOType=Inport  DeviceType=0
  in_DigitalOutputPWM.OUT_20_PWM_DIAG : KIBES_Signal/KIBES_Signal  MBDS_LibraryBlock=on  DatabaseKey=221  SignalName=DigitalOutputPWM.OUT_20_PWM_DIAG  SymbolName=DigitalOutputPWM_OUT_20_PWM_DIAG_000221  DataType=uint16  Init=1  Slope=1  Bias=0  DataSize=1  fpDataType=uint16  BlockIOType=Inport  DeviceType=0
  in_DigitalOutputPWM.OUT_20_TD : KIBES_Signal/KIBES_Signal  MBDS_LibraryBlock=on  DatabaseKey=222  SignalName=DigitalOutputPWM.OUT_20_TD  SymbolName=DigitalOutputPWM_OUT_20_TD_000222  DataType=boolean  Init=0  Slope=1  Bias=0  DataSize=1  fpDataType=boolean  BlockIOType=Inport  DeviceType=0
  in_DigitalOutputPWM.OUT_20_TD_DIAG : KIBES_Signal/KIBES_Signal  MBDS_LibraryBlock=on  DatabaseKey=223  SignalName=DigitalOutputPWM.OUT_20_TD_DIAG  SymbolName=DigitalOutputPWM_OUT_20_TD_DIAG_000223  DataType=uint16  Init=1  Slope=1  Bias=0  DataSize=1  fpDataType=uint16  BlockIOType=Inport  DeviceType=0
  in_DigitalOutputsSTATIC.OUT_01_TD : KIBES_Signal/KIBES_Signal  MBDS_LibraryBlock=on  DatabaseKey=217  SignalName=DigitalOutputsSTATIC.OUT_01_TD  SymbolName=DigitalOutputsSTATIC_OUT_01_TD_000217  DataType=boolean  Init=0  Slope=1  Bias=0  DataSize=1  fpDataType=boolean  BlockIOType=Inport  DeviceType=0
  in_DigitalOutputsSTATIC.OUT_01_TD_DIAG : KIBES_Signal/KIBES_Signal  MBDS_LibraryBlock=on  DatabaseKey=263  SignalName=DigitalOutputsSTATIC.OUT_01_TD_DIAG  SymbolName=DigitalOutputsSTATIC_OUT_01_TD_DIAG_000263  DataType=uint16  Init=1  Slope=1  Bias=0  DataSize=1  fpDataType=uint16  BlockIOType=Inport  DeviceType=0
  in_DigitalOutputsSTATIC.OUT_04_DIAG : KIBES_Signal/KIBES_Signal  MBDS_LibraryBlock=on  DatabaseKey=229  SignalName=DigitalOutputsSTATIC.OUT_04_DIAG  SymbolName=DigitalOutputsSTATIC_OUT_04_DIAG_000229  DataType=uint16  Init=1  Slope=1  Bias=0  DataSize=1  fpDataType=uint16  BlockIOType=Inport  DeviceType=0
  in_DigitalOutputsSTATIC.OUT_04_TD : KIBES_Signal/KIBES_Signal  MBDS_LibraryBlock=on  DatabaseKey=230  SignalName=DigitalOutputsSTATIC.OUT_04_TD  SymbolName=DigitalOutputsSTATIC_OUT_04_TD_000230  DataType=boolean  Init=0  Slope=1  Bias=0  DataSize=1  fpDataType=boolean  BlockIOType=Inport  DeviceType=0
  in_DigitalOutputsSTATIC.OUT_04_TD_DIAG : KIBES_Signal/KIBES_Signal  MBDS_LibraryBlock=on  DatabaseKey=231  SignalName=DigitalOutputsSTATIC.OUT_04_TD_DIAG  SymbolName=DigitalOutputsSTATIC_OUT_04_TD_DIAG_000231  DataType=uint16  Init=1  Slope=1  Bias=0  DataSize=1  fpDataType=uint16  BlockIOType=Inport  DeviceType=0
  in_STIMD.OUT_TdActivation : KIBES_Signal/KIBES_Signal  MBDS_LibraryBlock=on  DatabaseKey=225  SignalName=STIMD.OUT_TdActivation  SymbolName=STIMD_OUT_TdActivation_000225  DataType=boolean  Init=0  Slope=1  Bias=0  DataSize=1  fpDataType=boolean  BlockIOType=Inport  DeviceType=2
  in_STIMD.OUT_enable : KIBES_Signal/KIBES_Signal  MBDS_LibraryBlock=on  DatabaseKey=227  SignalName=STIMD.OUT_enable  SymbolName=STIMD_OUT_enable_000227  DataType=boolean  Init=0  Slope=1  Bias=0  DataSize=1  fpDataType=boolean  BlockIOType=Inport  DeviceType=2
  in_STIMD.OUT_value : KIBES_Signal/KIBES_Signal  MBDS_LibraryBlock=on  DatabaseKey=226  SignalName=STIMD.OUT_value  SymbolName=STIMD_OUT_value_000226  DataType=uint8  Init=0  Slope=1  Bias=0  DataSize=1  fpDataType=uint8  BlockIOType=Inport  DeviceType=2
  out_DigitalOutputPWM.OUT_20_PWM : KIBES_Signal/KIBES_Signal  MBDS_LibraryBlock=on  DatabaseKey=220  SignalName=DigitalOutputPWM.OUT_20_PWM  SymbolName=DigitalOutputPWM_OUT_20_PWM_000220  DataType=uint8  Init=0  Slope=1  Bias=0  DataSize=1  fpDataType=uint8  BlockIOType=Outport  DeviceType=0
  out_DigitalOutputPWM.OUT_20_TD_START : KIBES_Signal/KIBES_Signal  MBDS_LibraryBlock=on  DatabaseKey=224  SignalName=DigitalOutputPWM.OUT_20_TD_START  SymbolName=DigitalOutputPWM_OUT_20_TD_START_000224  DataType=boolean  Init=0  Slope=1  Bias=0  DataSize=1  fpDataType=boolean  BlockIOType=Outport  DeviceType=0
  out_DigitalOutputsSTATIC.OUT_01_TD_START : KIBES_Signal/KIBES_Signal  MBDS_LibraryBlock=on  DatabaseKey=219  SignalName=DigitalOutputsSTATIC.OUT_01_TD_START  SymbolName=DigitalOutputsSTATIC_OUT_01_TD_START_000219  DataType=boolean  Init=0  Slope=1  Bias=0  DataSize=1  fpDataType=boolean  BlockIOType=Outport  DeviceType=0
  out_DigitalOutputsSTATIC.OUT_04 : KIBES_Signal/KIBES_Signal  MBDS_LibraryBlock=on  DatabaseKey=228  SignalName=DigitalOutputsSTATIC.OUT_04  SymbolName=DigitalOutputsSTATIC_OUT_04_000228  DataType=boolean  Init=0  Slope=1  Bias=0  DataSize=1  fpDataType=boolean  BlockIOType=Outport  DeviceType=0
  out_DigitalOutputsSTATIC.OUT_04_TD_START : KIBES_Signal/KIBES_Signal  MBDS_LibraryBlock=on  DatabaseKey=232  SignalName=DigitalOutputsSTATIC.OUT_04_TD_START  SymbolName=DigitalOutputsSTATIC_OUT_04_TD_START_000232  DataType=boolean  Init=0  Slope=1  Bias=0  DataSize=1  fpDataType=boolean  BlockIOType=Outport  DeviceType=0
  out_OUT_DigitalOutputsSTATIC.OUT_01 : KIBES_Signal/KIBES_Signal  MBDS_LibraryBlock=on  DatabaseKey=81  SignalName=OUT_DigitalOutputsSTATIC.OUT_01  SymbolName=OUT_DigitalOutputsSTATIC_OUT_01_000081  DataType=boolean  Init=0  Slope=1  Bias=0  DataSize=1  fpDataType=boolean  BlockIOType=Outport  DeviceType=0
  wires:
  Data Type Conversion/1 -> out_OUT_DigitalOutputsSTATIC.OUT_01/1, out_DigitalOutputsSTATIC.OUT_04/1
  Switch1/1 -> out_DigitalOutputsSTATIC.OUT_01_TD_START/1, out_DigitalOutputPWM.OUT_20_TD_START/1, out_DigitalOutputsSTATIC.OUT_04_TD_START/1
  in_STIMD.OUT_TdActivation/1 -> Switch1/1
  Constant1/1 -> Switch1/3
  Switch/1 -> Data Type Conversion/1, out_DigitalOutputPWM.OUT_20_PWM/1
  in_STIMD.OUT_value/1 -> Switch/1
  Constant8/1 -> Switch/3
  in_STIMD.OUT_enable/1 -> Switch/2, Switch1/2
